simulink model "Engine_start_stop"  (R2014a)
settings: Solver=ode45  StartTime=0.0  StopTime=10.0  RelTol=1e-3
undefined symbols (not defined in the file): sigbuilder_block
settings Model: Creator=hemant6043  LastModifiedBy=hemant6043

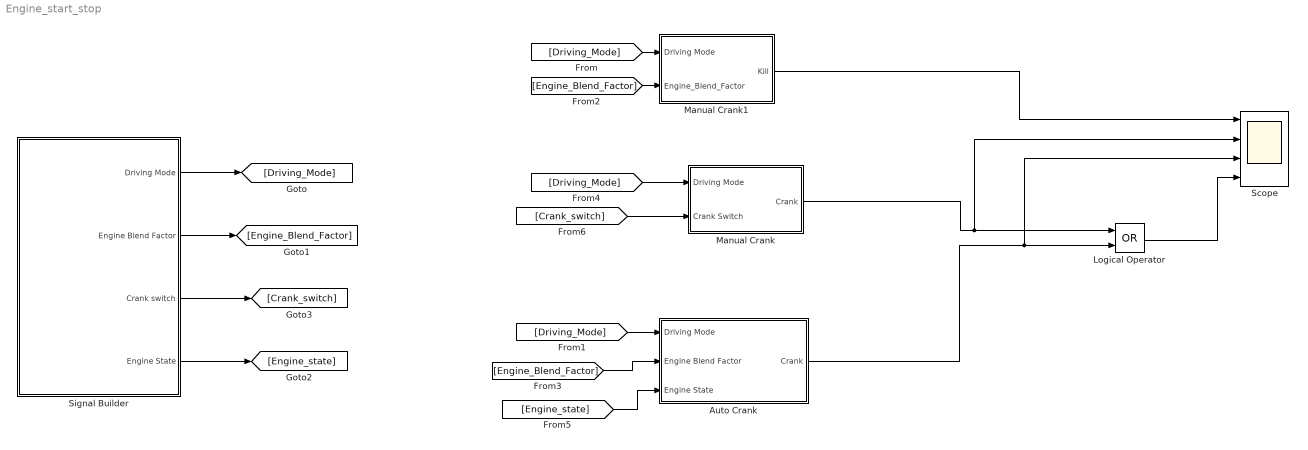
== system Engine_start_stop ==
  Auto Crank : Subsystem
  Logical Operator : Logic  Operator=OR  AllPortsSameDT=off  OutDataTypeStr=boolean
  Manual Crank : Subsystem
  Manual Crank1 : Subsystem
  Scope : Scope  NumInputPorts=4
      settings: YMin=-5~-5~-5~-5  YMax=5~5~5~5
  Signal Builder : Subsystem  Tag=STV Subsys  LoadFcn=sigbuilder_block('load',[68.25 -97.5 747 477.75 ]);  StartFcn=sigbuilder_block('start');  StopFcn=sigbuilder_block('stop');  ClipboardFcn=sigbuilder_block('clipboard');  mask(Sigbuilder block){}
      mask help: Simulink:masks:SigbuilderBlock_MD
      mask init:
      | if ~strcmp(get_param(bdroot(gcbh),'SimulationStatus'),'stopped') tuvar = sigbuilder_block('maskInit'); end
      settings: CopyFcn=sigbuilder_block('copy');  DeleteFcn=sigbuilder_block('delete');  ModelCloseFcn=sigbuilder_block('modelClose');  PreSaveFcn=sigbuilder_block('preSave');  PauseFcn=sigbuilder_block('pause');  ContinueFcn=sigbuilder_block('continue');  NameChangeFcn=sigbuilder_block('namechange');  OpenFcn=sigbuilder_block('open',[0 -228 1440 695.25 ]);  CloseFcn=sigbuilder_block('close');
      mask Display: plot(0, 0, 100, 100,[2, 2, 32, 32, 2], [68, 8, 8, 68, 68],[32, 2], [38, 38], [32, 19, 2],[53, 60, 44], [32, 17, 17, 2],[16, 16, 31, 31]);txt = getActiveGroup(gcbh);text(2, 100, txt,'verticalAlignment', 'top');
  wires:
  [Crank_switch] -> Manual Crank/2(Crank Switch)
  [Engine_state] -> Auto Crank/3(Engine State)
  Manual Crank1/1(Kill) -> Scope/1
  [Driving_Mode] -> Manual Crank1/1(Driving Mode)
  [Driving_Mode] -> Auto Crank/1(Driving Mode)
  [Engine_Blend_Factor] -> Manual Crank1/2(Engine_Blend_Factor)
  [Engine_Blend_Factor] -> Auto Crank/2(Engine Blend Factor)
  [Driving_Mode] -> Manual Crank/1(Driving Mode)
  Manual Crank/1(Crank) -> Scope/2, Logical Operator/1
  Logical Operator/1 -> Scope/4
  Signal Builder/1(Driving Mode) -> [Driving_Mode]
  Signal Builder/2(Engine Blend Factor) -> [Engine_Blend_Factor]
  Signal Builder/3(Crank switch) -> [Crank_switch]
  Signal Builder/4(Engine State) -> [Engine_state]
  Auto Crank/1(Crank) -> Scope/3, Logical Operator/2

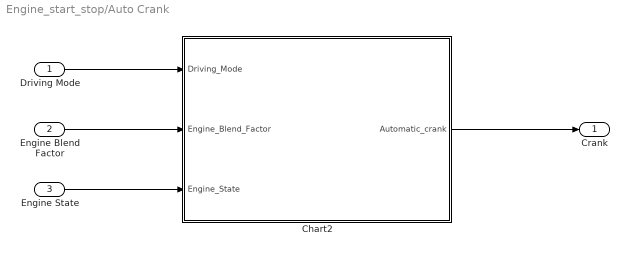
== system Engine_start_stop/Auto Crank ==
  Driving Mode : Inport
  Engine Blend Factor : Inport  Port=2
  Engine State : Inport  Port=3
  Chart2 : Stateflow chart  TreatAsAtomicUnit=on
  Crank : Outport
  wires:
  Chart2/1(Automatic_crank) -> Crank/1
  Engine State/1 -> Chart2/3(Engine_State)
  Engine Blend Factor/1 -> Chart2/2(Engine_Blend_Factor)
  Driving Mode/1 -> Chart2/1(Driving_Mode)

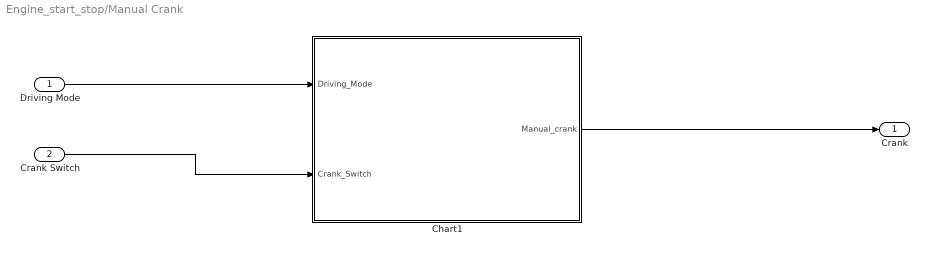
== system Engine_start_stop/Manual Crank ==
  Driving Mode : Inport
  Crank Switch : Inport  Port=2
  Chart1 : Stateflow chart  TreatAsAtomicUnit=on
  Crank : Outport
  wires:
  Driving Mode/1 -> Chart1/1(Driving_Mode)
  Crank Switch/1 -> Chart1/2(Crank_Switch)
  Chart1/1(Manual_crank) -> Crank/1

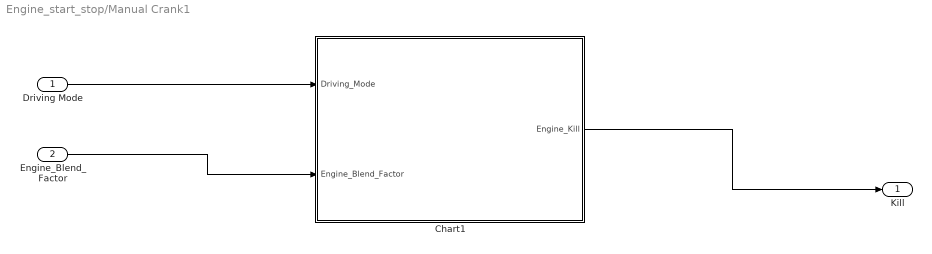
== system Engine_start_stop/Manual Crank1 ==
  Driving Mode : Inport
  Engine_Blend_Factor : Inport  Port=2
  Chart1 : Stateflow chart  TreatAsAtomicUnit=on
  Kill : Outport
  wires:
  Engine_Blend_Factor/1 -> Chart1/2(Engine_Blend_Factor)
  Driving Mode/1 -> Chart1/1(Driving_Mode)
  Chart1/1(Engine_Kill) -> Kill/1

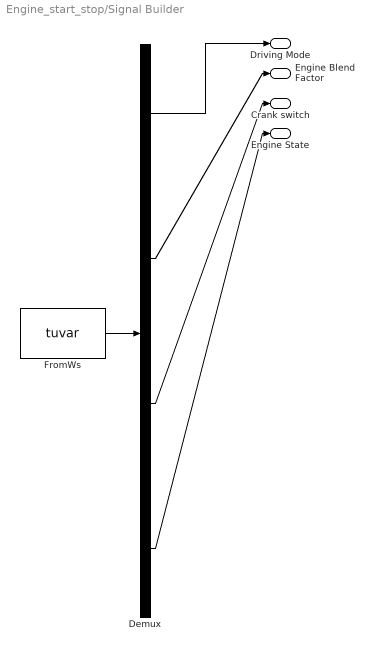
== system Engine_start_stop/Signal Builder ==
  Demux : Demux  Tag=STV Demux
  FromWs : FromWorkspace  Tag=STV FromWs  VariableName=tuvar  SampleTime=0
      SigBuilderData=|
      | common.afterFinalStr = 'Extrapolate'
      | common.sampleTime = 0
      | dataSet.timeRange = [0 10]
      | dataSet.name = 'Group 1'
      | sbobj.Groups.Name = 'Group 1'
      | sbobj.Groups.Signals(1).Name = 'Driving Mode'
      | sbobj.Groups.Signals(1).XData = [0 1 1 2.01 2.01 4 4 6 6 7 7 10]
      | sbobj.Groups.Signals(1).YData = [1 1 2 2 3 3 2 2 1 1 3 3]
      | sbobj.Groups.Signals(2).Name = 'Engine Blend Factor'
      | sbobj.Groups.Signals(2).XData = [0 3 3 5 5 10]
      | sbobj.Groups.Signals(2).YData = [0 0 0.02 0.02 0 0]
      | sbobj.Groups.Signals(3).Name = 'Crank switch'
      | sbobj.Groups.Signals(3).XData = [0 1 1 2 2 4 6 8.02 8.02 10]
      | sbobj.Groups.Signals(3).YData = [0 0 1 1 0 0 0 0 1 1]
      | sbobj.Groups.Signals(4).Name = 'Engine State'
      | sbobj.Groups.Signals(4).XData = [0 4 4 6 6 10]
      | sbobj.Groups.Signals(4).YData = [0 0 1 1 0 0]
  Driving Mode : Outport  Tag=STV Outport
  Engine Blend Factor : Outport  Tag=STV Outport  Port=2
  Crank switch : Outport  Tag=STV Outport  Port=3
  Engine State : Outport  Tag=STV Outport  Port=4
  wires:
  Demux/1 -> Driving Mode/1
  FromWs/1 -> Demux/1
  Demux/2 -> Engine Blend Factor/1
  Demux/3 -> Crank switch/1
  Demux/4 -> Engine State/1

== stateflow chart Engine_start_stop/Manual Crank/Chart1 ==
  state CRANK_ON
    during: Manual_crank=1
  state CRANKOFF
    during: Manual_crank=0
  CRANK_ON -> CRANKOFF : [Driving_Mode==1||Driving_Mode==2]
  CRANKOFF -> CRANK_ON : [Crank_Switch==1&&Driving_Mode==3]
  (default) -> CRANKOFF
  data: Driving_Mode input; Crank_Switch input; Manual_crank output

== stateflow chart Engine_start_stop/Auto Crank/Chart2 ==
  state CRANK_ON
    during: Automatic_crank=1
  state CRANKOFF
    during: Automatic_crank=0
  CRANK_ON -> CRANKOFF [order 1] : [Driving_Mode==1||Driving_Mode==3]
  CRANK_ON -> CRANKOFF [order 2] : [Driving_Mode==2&&Engine_Blend_Factor<0.01]
  CRANKOFF -> CRANK_ON : [Driving_Mode==2&&Engine_Blend_Factor>0.01&&Engine_State==1]
  (default) -> CRANKOFF
  data: Driving_Mode input; Engine_Blend_Factor input; Automatic_crank output; Engine_State input

== stateflow chart Engine_start_stop/Manual Crank1/Chart1 ==
  state KILL_ON
    during: Engine_Kill=1
  state KILL_OFF
    during: Engine_Kill=0
  KILL_ON -> KILL_OFF [order 2] : [Driving_Mode==2&&Engine_Blend_Factor>0.01]
  KILL_ON -> KILL_OFF [order 1] : [Driving_Mode==3]
  KILL_OFF -> KILL_ON [order 1] : [Driving_Mode==1]
  KILL_OFF -> KILL_ON [order 2] : [Driving_Mode==2&&Engine_Blend_Factor<0.01]
  (default) -> KILL_OFF
  data: Driving_Mode input; Engine_Blend_Factor input; Engine_Kill output
